simulink model "Part2_II"  (R2023b)
settings: Solver=VariableStepAuto  StartTime=0.0  StopTime=1  RelTol=1e-3
libraries: commrandsrc3 x1, commfilt2 x1
settings Model: Creator=henry  LastModifiedBy=henry

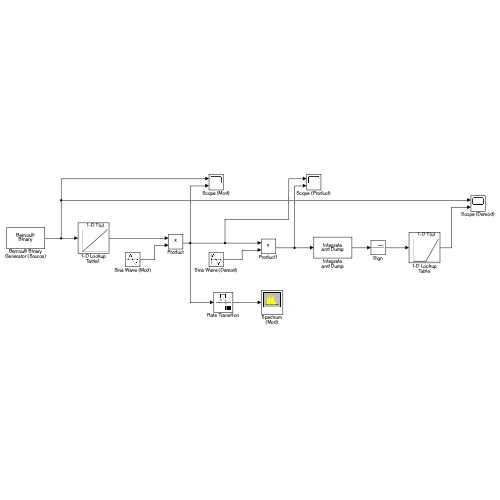
[thumbnail: Simulink's stored preview of the top-level diagram]
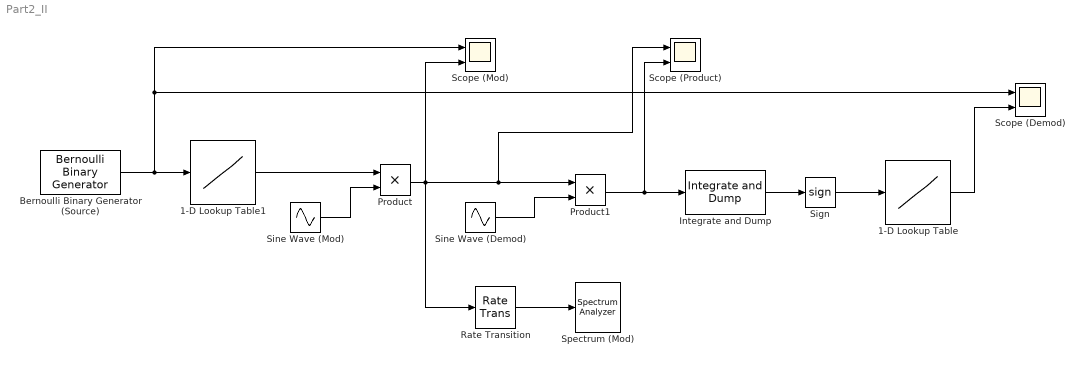
== system Part2_II ==
  1-D Lookup Table : Lookup_n-D  NumberOfTableDimensions=1  BreakpointsForDimension1=[-1,0,1]  Table=[0,0,1]  InternalRulePriority=Speed  RndMeth=Simplest
  1-D Lookup Table1 : Lookup_n-D  NumberOfTableDimensions=1  BreakpointsForDimension1=[0,1]  Table=[-1,1]  InternalRulePriority=Speed  RndMeth=Simplest
  Bernoulli Binary Generator (Source) : commrandsrc3/Bernoulli Binary Generator  ProbabilityOfZero=0.5  SeedSource=Parameter  Seed=100  SampleTime=0.001  SamplesPerFrame=1  OutputDataType=double  SimulateUsing=Interpreted execution
  Integrate and Dump : commfilt2/Integrate and Dump  obssamples=8  offsetsamples=0  nodump=off  roundingMode=Floor  overflowMode=off  outputDataTypeStr=Inherit: Same as accumulator  outputLastDataTypeStr=Inherit: Same as accumulator
  Product : Product
  Product1 : Product
  Rate Transition : RateTransition  OutPortSampleTime=0.5e-4
  Scope (Demod) : Scope  NumInputPorts=2
  Scope (Mod) : Scope  NumInputPorts=2
  Scope (Product) : Scope  NumInputPorts=2
  Sign : Signum
  Sine Wave (Demod) : Sin  SineType=Sample based  Samples=5000  SampleTime=1e-7
  Sine Wave (Mod) : Sin  SineType=Sample based  Samples=5000  SampleTime=1e-7
  Spectrum (Mod) : SpectrumAnalyzer  WindowPosition=[320.000000,200.000000,800.000000,500.000000,]  Visible=on  ScopeFrameLocation=window  Span=20000  StartFrequency=-10000  StopFrequency=10000  YLimits=[-71.15518083,16.16696979]
  wires:
  Bernoulli Binary Generator (Source)/1 -> Scope (Demod)/1, Scope (Mod)/1, 1-D Lookup Table1/1
  Sine Wave (Mod)/1 -> Product/2
  Product/1 -> Scope (Product)/1, Product1/1, Rate Transition/1, Scope (Mod)/2
  Rate Transition/1 -> Spectrum (Mod)/1
  Sine Wave (Demod)/1 -> Product1/2
  Product1/1 -> Scope (Product)/2, Integrate and Dump/1
  Integrate and Dump/1 -> Sign/1
  Sign/1 -> 1-D Lookup Table/1
  1-D Lookup Table/1 -> Scope (Demod)/2
  1-D Lookup Table1/1 -> Product/1
